simulink model "Washing_Machine"  (R2024b)
settings: Solver=VariableStepAuto  StartTime=0.0  StopTime=100.0  RelTol=1e-3

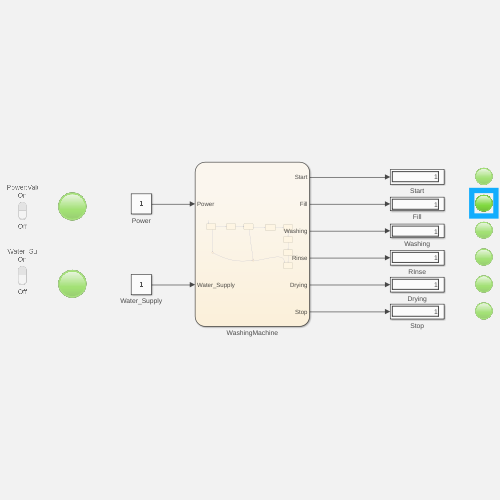
[thumbnail: Simulink's stored preview of the top-level diagram]
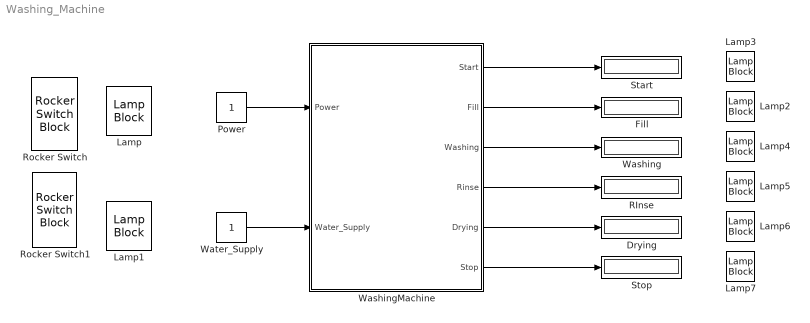
== system Washing_Machine ==
  Drying : Display
  Fill : Display
  Lamp{,1..7} (8 alike) : LampBlock  LabelPosition=Hide
  Power : Constant
  RInse : Display
  Rocker Switch : RockerSwitchBlock
      settings: Values={{'Off', 'On'}, [0 1]}
  Rocker Switch1 : RockerSwitchBlock
      settings: Values={{'Off', 'On'}, [0 1]}
  Start : Display
  Stop : Display
  Washing : Display
  WashingMachine : Stateflow chart  TreatAsAtomicUnit=on
  Water_Supply : Constant
  wires:
  WashingMachine/1(Start) -> Start/1
  WashingMachine/6(Stop) -> Stop/1
  WashingMachine/3(Washing) -> Washing/1
  WashingMachine/4(Rinse) -> RInse/1
  WashingMachine/5(Drying) -> Drying/1
  Power/1 -> WashingMachine/1(Power)
  Water_Supply/1 -> WashingMachine/2(Water_Supply)
  WashingMachine/2(Fill) -> Fill/1

== stateflow chart Washing_Machine/WashingMachine ==
  state ON
    entry:
    Start=1
  state Water_Supply
  state Power
  state Fill
    entry:
    Fill=1
  state Washing
    entry:
    Washing=1
  state RInse
    entry:
    Rinse=1
  state Drying
    entry:
    Drying=1
  state OFF
    entry:
    Stop=1
  (default) -> Power
  Power -> ON [order 1] : {Power==1}
  ON -> Water_Supply
  Water_Supply -> Fill [order 1] : [Water_Supply==1]
  Fill -> Washing : [after(20,sec)]
  Power -> (junction 17) [order 2] : [Power==0]
  Water_Supply -> (junction 18) [order 2] : [Water_Supply==0]
  Washing -> RInse : [after(10,sec)]
  RInse -> Drying : [after(20,sec)]
  (junction 17) -> (junction 18)
  Drying -> OFF : [after(15,sec)]
  (junction 18) -> OFF
  data: Start output; Fill output; Power input; Water_Supply input; Washing output; Rinse output; Drying output; Stop output
